simulink model "pid_controller_pitch"  (R2023a)
settings: Solver=FixedStepAuto  StartTime=0.0  StopTime=inf  FixedStep=Ts_slk  RelTol=1e-3  EnableMultiTasking=on
undefined symbols (not defined in the file): A_cond, B_cond, C, D, dev, IMU_w_b_bias, K, Main, meas_pole, P0_phth, P0_ps, prefilter_pole, pwm_output0, Q_phth, q_ps, R_phth, r_ps, Rz, Ts_EKF_integr, Ts_EKF_meas, Ts_slk, x0_phth, x0_ps
libraries: px4Sensorslib x4, slpidlib x2, cstblocks x1, px4lib x1, px4uORBlib x1, sharedtransform x1
(part 2 of 2)

== matlab function pid_controller_pitch/Observer/unlimited RPY/unlimited RPY ==
  data: RPY input; RPY output; RPY1 input; init output; init input
function [RPY,init] = unlimited_RPY(RPY,RPY1, init)
if init == 0
    init = 1;
    RPY1 = RPY;
end

for i =1:1:3
    while abs(RPY(i) - RPY1(i)) > pi/2
        RPY(i) = RPY(i) + sign(RPY1(i))*pi;
    end
end
end

== matlab function pid_controller_pitch/Observer/Subsystem/MATLAB Function7 ==
  data: u input; y1 output; y2 output; y3 output
function [y1,y2,y3] = fcn(u)

y1 = u(1);
y2 = u(2);
y3 = u(3);

== matlab function pid_controller_pitch/unlimited RPY2/unlimited RPY ==
  data: RPY input; RPY output; RPY1 input; init output; init input
function [RPY,init] = unlimited_RPY(RPY,RPY1, init)
if init == 0
    init = 1;
    RPY1 = RPY;
end

for i =1:1:3
    while abs(RPY(i) - RPY1(i)) > pi/2
        RPY(i) = RPY(i) + sign(RPY1(i))*pi;
    end
end
end

== matlab function pid_controller_pitch/Observer/Subsystem/unlimited RPY1/unlimited RPY ==
  data: RPY input; RPY output; RPY1 input; init output; init input
function [RPY,init] = unlimited_RPY(RPY,RPY1, init)
if init == 0
    init = 1;
    RPY1 = RPY;
end

for i =1:1:3
    while abs(RPY(i) - RPY1(i)) > pi/2
        RPY(i) = RPY(i) + sign(RPY1(i))*pi;
    end
end
end

== matlab function pid_controller_pitch/Observer/Subsystem/MATLAB Function1 ==
  data: u input; y1 output; y2 output; y3 output
function [y1,y2,y3] = fcn(u)

y1 = u(1);
y2 = u(2);
y3 = u(3);

== matlab function pid_controller_pitch/Controller Karimi 2105/MATLAB Function3 ==
  data: tau input; tau_o output
function tau_o=fcn(tau)
% Inputs:   tau    (torque 1x1)         
%
% Outputs:  tau_o  (torque 3x1)

% States in input
tau_1     =       tau(1,1);     %  roll torque

% States in output
tau_o      =       zeros(3,1);
tau_o(1,1) =       tau_1;   
tau_o(2,1) =       0;
tau_o(3,1) =       0;

== matlab function pid_controller_pitch/Observer/IMU measurements & rotation/MATLAB Function1 ==
  data: u input; y output
function y = w_b_roation(u)
y = zeros(3,1);
y(1) = +u(1);
y(2) = -u(2);
y(3) = -u(3);
end

== matlab function pid_controller_pitch/Observer/Observer/Y_computation ==
  data: mf_b input; RP_estim input; Y_meas output
function Y_meas    = Y_computation(mf_b,RP_estim)
% description:
% - a_b             = measured linear acceleration in body-frame
% - w_b             = measured angular velocity in body-frame
% - mf_b            = measured magnetic field in body-frame
% - mf              = measured magnetic field in body-inertia
% - a_b_disturbe    = linear velocity measurement-noise
% - w_b_disturbe    = angular velocity measurement-noise
% - mf_b_disturbe   = magnetic field measurement-noise

% -------------------------------------------------------------------------------------------
% observation: the following computation works only if the angles
% phi,theta,psy are withing angles (-pi/2,+pi/2) (this is an open set, pi/2 is excluded)
% -------------------------------------------------------------------------------------------

ph_estim = RP_estim(1,1);
th_estim = RP_estim(2,1);

sph = sin(ph_estim);
cph = cos(ph_estim);

sth = sin(th_estim);
cth = cos(th_estim);

ps_meas_num   = mf_b(3)*sph - mf_b(2)*cph;
ps_meas_den = mf_b(1)*cth + mf_b(2)*sth*sph + mf_b(3)*sth*cph;
ps_meas = atan2(ps_meas_num, ps_meas_den);

if ps_meas < 0
    ps_meas = ps_meas + 2*pi;
end

Y_meas = ps_meas;
end

== matlab function pid_controller_pitch/Observer/Observer/Y_EKF/EKF_Y ==
  data: time input; xk1 input size=[1,1]; Pk1 input size=[1,1]; w_b1 input; Y_meas input; RP_estim input; bias_w_b_estim input; t_meas input; q_ps parameter; xk output size=[1,1]; Pk output; t_meas output; r_ps parameter; Ts_EKF_integr parameter; Ts_EKF_meas parameter
function [xk,Pk,t_meas] = EKF_Y(time,xk1,Pk1,w_b1,Y_meas,RP_estim,bias_w_b_estim,t_meas,q_ps,r_ps,Ts_EKF_integr,Ts_EKF_meas)

if time - t_meas >= Ts_EKF_meas
    t_meas = time;
    Q = q_ps;
    R = r_ps;

  % INTEGRATION STEP
    % initial condition
    xt1         =       xk1;                        % initial condition for the state
    Pt1         =       Pk1;                        % initial condition for matrix P

    wp1         =       w_b1(1,1);                  % past value of the p-dir of angular velocity w
    wq1         =       w_b1(2,1);                  % past value of the q-dir of angular velocity w
    wr1         =       w_b1(3,1);                  % past value of the r-dir of angular velocity w

    phi         =       RP_estim(1,1);              % estimate of roll angle (rad)
    theta       =       RP_estim(2,1);              % estimate of pitch angle (rad)  

    bias_wp     =       bias_w_b_estim(1,1);        % estimate of bias of p-dir of angular velocity w
    bias_wq     =       bias_w_b_estim(2,1);        % estimate of bias of q-dir of angular velocity w
    bias_wr     =       bias_w_b_estim(3,1);        % estimate of bias of r-dir of angular velocity w
    % integration loop
    Nstep       = floor(Ts_EKF_meas/Ts_EKF_integr); % number of integration steps to performe in the t_meas time windows
    xt          = zeros(1,1);
    Pt          = zeros(1,1);
    for i = 1:1:Nstep
        % state extraction
            psi         =       xt1(1,1);           % roll angle (rad)
        
            cph         =       cos(phi);
            cth         =       cos(theta);
            cps         =       cos(psi);
            sph         =       sin(phi);
            sth         =       sin(theta);
            sps         =       sin(psi);
            tth         =       sth/cth;
        % integration
            Mf = [0,    sph/cth,    cph/cth,    0,  0,  0;];
            Z1 = [wp1-bias_wp; wq1-bias_wq; wr1-bias_wr; bias_wp; bias_wq; bias_wr;];
            f = Mf*Z1;
            xt = xt1 + Ts_EKF_integr*f;
        
            At1 = 0;
            Pt = Pt1 + Ts_EKF_integr*(At1*Pt1 + Pt1*At1' + Q);
        % house keeping
            xt1 = xt;
            Pt1 = Pt;
    end
  % MEASUREMENT STEP
    Ck = [eye(1)];
    Lk = Pt*Ck'/(Ck*Pt*Ck' + R);
    xk = xt + Lk*(Y_meas - Ck*xt);
    Pk = (eye(1) - Lk*Ck)*Pt;
else
    xk = xk1;
    Pk = Pk1;
end
end

== matlab function pid_controller_pitch/Observer/Observer/RP_computation ==
  data: a_b input; RP_meas output
function RP_meas    = RP_computation(a_b)
% description:
% - a_b             = measured linear acceleration in body-frame
% - w_b             = measured angular velocity in body-frame
% - mf_b            = measured magnetic field in body-frame
% - mf              = measured magnetic field in body-inertia
% - a_b_disturbe    = linear velocity measurement-noise
% - w_b_disturbe    = angular velocity measurement-noise
% - mf_b_disturbe   = magnetic field measurement-noise

% -------------------------------------------------------------------------------------------
% observation: the following computation works only if the angles
% phi,theta,psy are withing angles (-pi/2,+pi/2) (this is an open set, pi/2 is excluded)
% -------------------------------------------------------------------------------------------

a_b = -1*a_b;       % need to adjust the sign to use atan2() function correctly

% phi computation
ph_meas = atan2(a_b(2), a_b(3));
sph = sin(ph_meas);
cph = cos(ph_meas);

% theta computation
th_meas = atan2(-a_b(1), (a_b(2)*sph + a_b(3)*cph));

RP_meas = [ph_meas;th_meas];

== matlab function pid_controller_pitch/Observer/Observer/RP_EKF/EKF_RP ==
  data: time input; xk1 input; Pk1 input; w_b1 input; RP_meas input; t_meas input; Q_phth parameter; xk output; Pk output; t_meas output; R_phth parameter; Ts_EKF_integr parameter; Ts_EKF_meas parameter
function [xk,Pk,t_meas] = EKF_RP(time,xk1,Pk1,w_b1,RP_meas,t_meas,Q_phth,R_phth,Ts_EKF_integr,Ts_EKF_meas)

if time - t_meas >= Ts_EKF_meas
    t_meas = time;
    Q = Q_phth;
    R = R_phth;

  % INTEGRATION STEP
    % initial condition
    xt1         =       xk1;                        % initial condition for the state
    Pt1         =       Pk1;                        % initial condition for matrix P
    wp1         =       w_b1(1,1);                  % past value of the p-dir of angular velocity w
    wq1         =       w_b1(2,1);                  % past value of the q-dir of angular velocity w
    wr1         =       w_b1(3,1);                  % past value of the r-dir of angular velocity w
    % integration loop
    Nstep       = floor(Ts_EKF_meas/Ts_EKF_integr); % number of integration steps to performe in the t_meas time windows
    xt          = zeros(5,1);
    Pt          = zeros(5,5);
    for i = 1:1:Nstep
        % state extraction
            phi         =       xt1(1,1);           % roll angle (rad)
            theta       =       xt1(2,1);           % pitch angle (rad)  
            bias_wp     =       xt1(3,1);           % bias of p-dir of angular velocity w
            bias_wq     =       xt1(4,1);           % bias of q-dir of angular velocity w
            bias_wr     =       xt1(5,1);           % bias of r-dir of angular velocity w
        
            cph         =       cos(phi);
            cth         =       cos(theta);
            sph         =       sin(phi);
            sth         =       sin(theta);
            tth         =       sth/cth;
        % integration
            Mf = [1,    sph*tth,    cph*tth,    0,  0,  0;
                  0,    cph,        -sph,       0,  0,  0;
                  0,    0,          0,          0,  0,  0;
                  0,    0,          0,          0,  0,  0;
                  0,    0,          0,          0,  0,  0;];
            Z1 = [wp1-bias_wp; wq1-bias_wq; wr1-bias_wr; bias_wp; bias_wq; bias_wr;];
            f = Mf*Z1;
            xt = xt1 + Ts_EKF_integr*f;
        
            A1 = [cph*tth*(wq1-bias_wq)-sph*tth*(wr1-bias_wr),(sph*(wq1-bias_wq)+cph*(wr1-bias_wr))/cth^2,  -1, -sph*tth,   -cph*tth;];
            A2 = [-sph*(wq1-bias_wq)-cph*(wr1-bias_wr),  0,  0,  -cph,   sph;];
            A3 = [0,  0,  0,  0,  0;];
            A4 = [0,  0,  0,  0,  0;];
            A5 = [0,  0,  0,  0,  0;];
            At1 = [A1; A2; A3; A4; A5;];
            Pt = Pt1 + Ts_EKF_integr*(At1*Pt1 + Pt1*At1' + Q);
        % house keeping
            xt1 = xt;
            Pt1 = Pt;
    end
  % MEASUREMENT STEP
    Ck = [eye(2),zeros(2,3)];
    Lk = Pt*Ck'/(Ck*Pt*Ck' + R);
    xk = xt + Lk*(RP_meas - Ck*xt);
    Pk = (eye(5) - Lk*Ck)*Pt;
else
    xk = xk1;
    Pk = Pk1;
end
end

== matlab function pid_controller_pitch/PX4/Acquisition/MATLAB Function ==
  data: u input; y1 output; y2 output; y3 output; y4 output; y5 output; y6 output
function [y1,y2,y3,y4,y5,y6] = fcn(u)

y1 = u(1);
y2 = u(2);
y3 = u(3);
y4 = u(4);
y5 = u(5);
y6 = u(6);
